simulink model "Bridge_simu_PP"  (R2022a)
settings: Solver=ode4  StartTime=t_init  StopTime=t_final  FixedStep=t_step  RelTol=1e-3
values from neighbouring files (symbols this model uses):
  x0 = [1/20; 1/100; 0; 0]    [MDOF_Pbridge_PP.m]
undefined symbols (not defined in the file or in its folder): As, Bs, Cs, Ds
settings Model: Creator=conni  LastModifiedBy=LEGION
settings DebuggingCC: UnconnectedInputMsg=warning  UnconnectedOutputMsg=warning  UnconnectedLineMsg=warning  SFMachineParentedDataDiag=warning
settings SFSimCC: CustomCodeUndefinedFunction=UseInterfaceOnly
settings RTWCC: DLArmComputeVersion=19.05

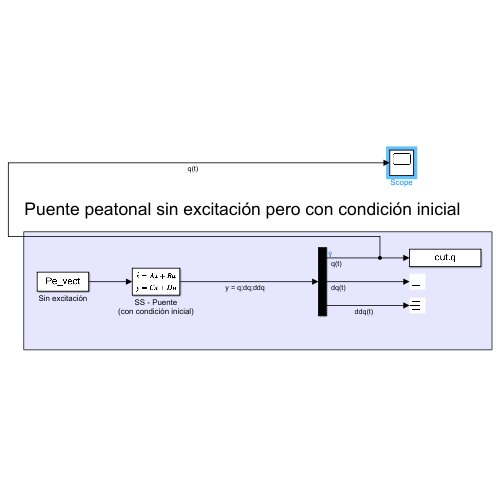
[thumbnail: Simulink's stored preview of the top-level diagram]
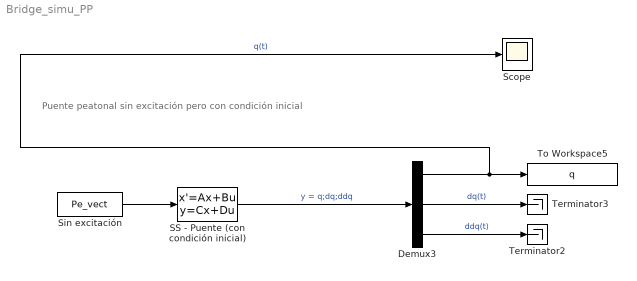
== system Bridge_simu_PP ==
  note: Puente peatonal sin excitación pero con condición inicial
  Demux3 : Demux  Outputs=3
  SS - Puente (con condición inicial) : StateSpace  A=As  B=Bs  C=Cs  D=Ds  InitialCondition=x0
  Scope : Scope
  Sin excitación : FromWorkspace  VariableName=Pe_vect
  Terminator2 : Terminator
  Terminator3 : Terminator
  To Workspace5 : ToWorkspace  VariableName=q  SaveFormat=Timeseries  SampleTime=-1
  wires:
  SS - Puente (con condición inicial)/1 -> Demux3/1  "y = q;dq;ddq"
  Demux3/1 -> Scope/1, To Workspace5/1  "q(t)"
  Demux3/2 -> Terminator3/1  "dq(t)"
  Demux3/3 -> Terminator2/1  "ddq(t)"
  Sin excitación/1 -> SS - Puente (con condición inicial)/1
